simulink subsystem "EncoderVelocidad"  (R2023b)
settings: Solver=VariableStepAuto  StartTime=0.0  StopTime=10.0  RelTol=1e-3
libraries: arduinosensorlib x2, simulink x1
settings Model: Creator=chaya  LastModifiedBy=chaya

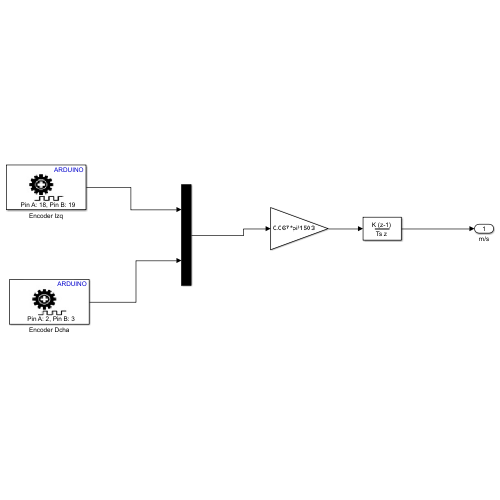
[thumbnail: Simulink's stored preview of the top-level diagram]
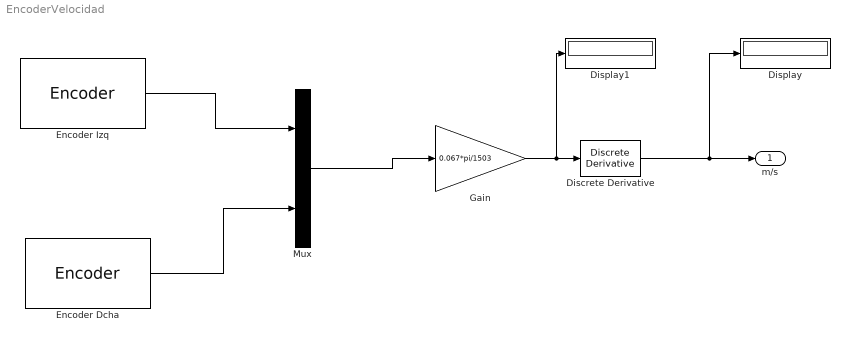
== system EncoderVelocidad ==
  Discrete Derivative : simulink/Discrete/Discrete Derivative  gainval=1.0  ICPrevScaledInput=0.0  OutMin=[]  OutMax=[]  OutDataTypeStr=double  OutputDataTypeScalingMode=double  OutDataType=fixdt(1, 16)  OutScaling=2^-10  DoSatur=off
  Display : Display
  Display1 : Display
  Encoder Dcha : arduinosensorlib/Encoder  InputA=2  InputB=3  Mode=No reset  SampleTime=0.01
  Encoder Izq : arduinosensorlib/Encoder  InputA=18  InputB=19  Mode=No reset  SampleTime=0.01
  Gain : Gain  Gain=0.067*pi/1503
  Mux : Mux  Inputs=2
  m/s : Outport
  wires:
  Discrete Derivative/1 -> m/s/1, Display/1
  Gain/1 -> Discrete Derivative/1, Display1/1
  Mux/1 -> Gain/1
  Encoder Dcha/1 -> Mux/2
  Encoder Izq/1 -> Mux/1
